simulink model "switchupg"  (R2020b)
settings: Solver=VariableStepAuto  StartTime=0.0  StopTime=10.0  RelTol=1e-3
libraries: fl_lib x5, ee_lib x3
settings Model: Creator=test  LastModifiedBy=test

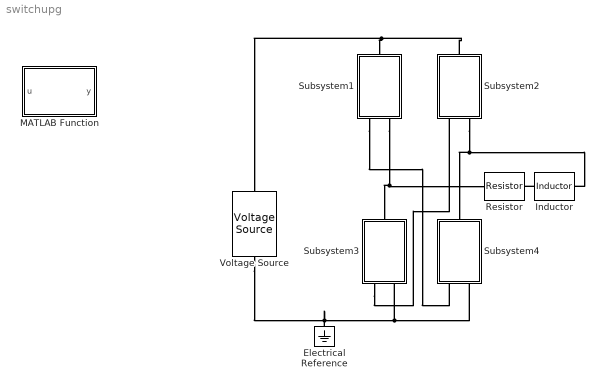
== system switchupg ==
  Electrical Reference : fl_lib/Electrical/Electrical Elements/Electrical Reference
  Inductor : ee_lib/Passive/Inductor  l=1e-6 H  L_tol=20  enable_L_tol=0  tol_distribution=1  nSigma=4  r=0 Ohm  g=1e-9 1/Ohm  enable_operating_limits=0  operating_limit_action=2  max_working_current=1 A  power_rating=1 W  enable_faults=0  fault_action=1  lambdaPercent=50  k_faulted=0.9999  turnsShort=0  openCct=0  groundShort=0  groundShortG=0 1/Ohm  tau_fault=1e-3 s  enable_temporal_fault=0  t_fault=1 s  enable_behavioral_fault=0  max_permissible_voltage=100 V  n_fail_on_voltage=1  max_permissible_current=1 A  t_fail_on_current=1 s  i_L_specify=off  i_L_priority=High  i_L=0 A  i_L_nominal_specify=off  i_L_nominal_unit=A  i_L_nominal_value=1
  MATLAB Function : MATLAB Function  TreatAsAtomicUnit=on
  Resistor : ee_lib/Passive/Resistor  R=1 Ohm  R_tol=5  enable_R_tol=0  tol_distribution=1  nSigma=4  enable_operating_limits=0  operating_limit_action=2  max_working_voltage=100 V  power_rating=1 W  enable_faults=0  fault_action=1  R_faulted=inf Ohm  enable_temporal_fault=0  t_fault=1 s  enable_behavioral_fault=0  max_permissible_current=1 A  t_fail_on_current=1 s  noise_mode=0  sample_time=1e-3 s  repeatability=1  auto_seed=3499211588  user_seed=0  Tdevice=25 degC  alpha=3.93e-3 1/K  Tmeas=25 degC  thermal_mass=100 J/K  power_derating_T1=70 degC  power_derating_T2=155 degC  operating_temperature_range_vec=[-50, 150] degC  temperature_specify=off  temperature_priority=High  temperature=298.15 K  temperature_nominal_specify=off  temperature_nominal_unit=K  temperature_nominal_value=1
  Subsystem1 : Subsystem
  Subsystem2 : Subsystem
  Subsystem3 : Subsystem
  Subsystem4 : Subsystem
  Voltage Source : ee_lib/Sources/Voltage Source  dc_voltage=10 V  ac_voltage=0 V  ac_shift=0 rad  ac_frequency=60 Hz  noise_mode=0  PSD=0 V^2/Hz  repeatability=1  auto_seed=3890346746  user_seed=0  sample_time=1e-3 s  i_specify=off  i_priority=None  i=0 A  i_nominal_specify=off  i_nominal_unit=A  i_nominal_value=1  v_specify=off  v_priority=None  v=0 V  v_nominal_specify=off  v_nominal_unit=V  v_nominal_value=1
  connections:
  Voltage Source/RConn1 -- Electrical Reference/LConn1 -- Subsystem4/RConn2 -- Subsystem3/RConn2
  Inductor/LConn1 -- Resistor/RConn1
  Subsystem2/LConn1 -- Subsystem1/LConn1 -- Voltage Source/LConn1
  Subsystem1/RConn1 -- Subsystem4/RConn1
  Subsystem3/RConn1 -- Subsystem2/RConn1
  Subsystem1/RConn2 -- Subsystem3/LConn1 -- Resistor/LConn1
  Subsystem2/RConn2 -- Subsystem4/LConn1 -- Inductor/RConn1

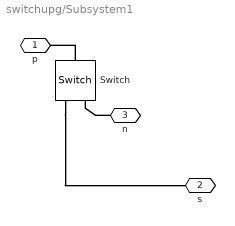
== system switchupg/Subsystem1 ==
  Switch : fl_lib/Electrical/Electrical Elements/Switch  R_closed=0.01 Ohm  G_open=1e-8 1/Ohm  Threshold=0.5  i_specify=off  i_priority=None  i=0 A  i_nominal_specify=off  i_nominal_unit=A  i_nominal_value=1  v_specify=off  v_priority=None  v=0 V  v_nominal_specify=off  v_nominal_unit=V  v_nominal_value=1
  p : PMIOPort  Side=Left
  s : PMIOPort  Port=2  Side=Right
  n : PMIOPort  Port=3  Side=Right
  connections:
  Switch/LConn1 -- p/RConn1
  n/RConn1 -- Switch/RConn2
  Switch/RConn1 -- s/RConn1

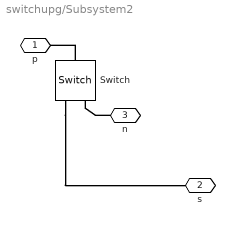
== system switchupg/Subsystem2 ==
  Switch : fl_lib/Electrical/Electrical Elements/Switch  R_closed=0.01 Ohm  G_open=1e-8 1/Ohm  Threshold=0.5  i_specify=off  i_priority=None  i=0 A  i_nominal_specify=off  i_nominal_unit=A  i_nominal_value=1  v_specify=off  v_priority=None  v=0 V  v_nominal_specify=off  v_nominal_unit=V  v_nominal_value=1
  p : PMIOPort  Side=Left
  s : PMIOPort  Port=2  Side=Right
  n : PMIOPort  Port=3  Side=Right
  connections:
  Switch/LConn1 -- p/RConn1
  n/RConn1 -- Switch/RConn2
  Switch/RConn1 -- s/RConn1

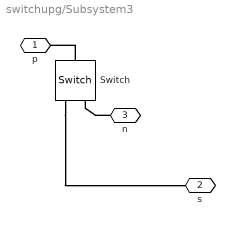
== system switchupg/Subsystem3 ==
  Switch : fl_lib/Electrical/Electrical Elements/Switch  R_closed=0.01 Ohm  G_open=1e-8 1/Ohm  Threshold=0.5  i_specify=off  i_priority=None  i=0 A  i_nominal_specify=off  i_nominal_unit=A  i_nominal_value=1  v_specify=off  v_priority=None  v=0 V  v_nominal_specify=off  v_nominal_unit=V  v_nominal_value=1
  p : PMIOPort  Side=Left
  s : PMIOPort  Port=2  Side=Right
  n : PMIOPort  Port=3  Side=Right
  connections:
  Switch/LConn1 -- p/RConn1
  n/RConn1 -- Switch/RConn2
  Switch/RConn1 -- s/RConn1

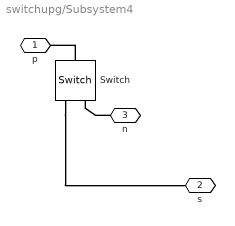
== system switchupg/Subsystem4 ==
  Switch : fl_lib/Electrical/Electrical Elements/Switch  R_closed=0.01 Ohm  G_open=1e-8 1/Ohm  Threshold=0.5  i_specify=off  i_priority=None  i=0 A  i_nominal_specify=off  i_nominal_unit=A  i_nominal_value=1  v_specify=off  v_priority=None  v=0 V  v_nominal_specify=off  v_nominal_unit=V  v_nominal_value=1
  p : PMIOPort  Side=Left
  s : PMIOPort  Port=2  Side=Right
  n : PMIOPort  Port=3  Side=Right
  connections:
  Switch/LConn1 -- p/RConn1
  n/RConn1 -- Switch/RConn2
  Switch/RConn1 -- s/RConn1

== matlab function switchupg/MATLAB Function ==
  data: u input; y output
function y = fcn(u)

y = u;
